simulink model "cascadecontrol"  (Simulink 6.0)
settings: Solver=ode45  StartTime=0.0  StopTime=1000  RelTol=1e-3
libraries: simulink_extras x3, simulink x1
settings Model: LastModifiedBy=lenovo

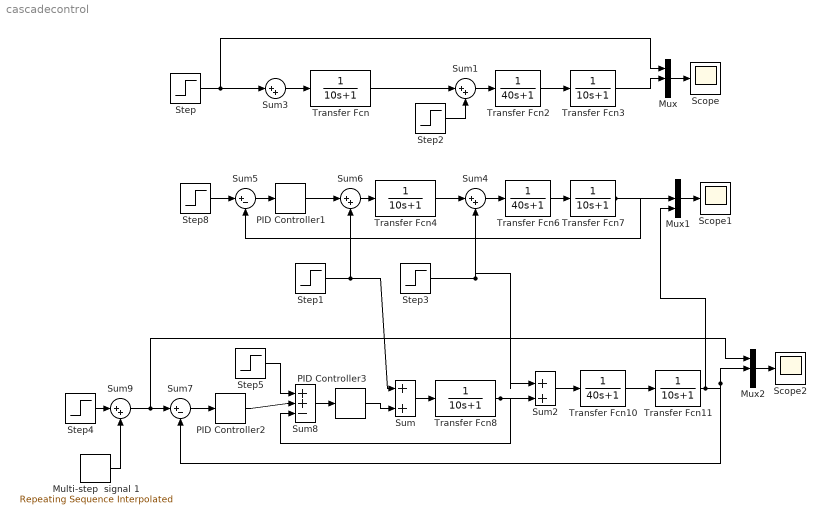
== system cascadecontrol ==
  Multi-step  signal 1 : simulink/Sources/Repeating Sequence Interpolated  OutValues=[1 2 1.5 1 1.5].'  TimeValues=[0 28 55 80 100]*10.'  LookUpMeth=Use Input Below  tsamp=1  OutputDataTypeScalingMode=Specify via dialog  OutDataType=float('double')  OutScaling=2^-10
  Mux : Mux  Inputs=3
  Mux1 : Mux  Inputs=3
  Mux2 : Mux  Inputs=3
  PID Controller1 : simulink_extras/Additional Linear/PID Controller  P=4  I=0.05  D=20
  PID Controller2 : simulink_extras/Additional Linear/PID Controller  P=10  I=0.15  D=45
  PID Controller3 : simulink_extras/Additional Linear/PID Controller  P=1.5  I=0  D=0
  Scope : Scope
  Scope1 : Scope
  Scope2 : Scope
      settings: SaveName=ScopeData2
  Step : Step  Time=0  SampleTime=0
  Step{1..5,8} (6 alike) : Step  Time=0  After=0  SampleTime=0
  Sum{,1..4,6,9} (7 alike) : Sum  Inputs=|++
  Sum5 : Sum  Inputs=|+-
  Sum7 : Sum  Inputs=|+-
  Sum8 : Sum  Inputs=|++-
  Transfer Fcn{,3..4,7..8,11} (6 alike) : TransferFcn  Denominator=[10 1]
  Transfer Fcn10 : TransferFcn  Denominator=[40 1]
  Transfer Fcn2 : TransferFcn  Denominator=[40 1]
  Transfer Fcn6 : TransferFcn  Denominator=[40 1]
  wires:
  Step/1 -> Mux/1, Sum3/1
  Transfer Fcn/1 -> Sum1/1
  Sum1/1 -> Transfer Fcn2/1
  Transfer Fcn3/1 -> Mux/2
  Mux/1 -> Scope/1
  Transfer Fcn2/1 -> Transfer Fcn3/1
  Sum5/1 -> PID Controller1/1
  PID Controller1/1 -> Sum6/1
  Sum4/1 -> Transfer Fcn6/1
  Transfer Fcn7/1 -> Sum5/2, Mux1/2
  Mux1/1 -> Scope1/1
  Sum6/1 -> Transfer Fcn4/1
  Transfer Fcn6/1 -> Transfer Fcn7/1
  Step2/1 -> Sum1/2
  Sum3/1 -> Transfer Fcn/1
  Step3/1 -> Sum4/2, Sum2/1
  Sum7/1 -> PID Controller2/1
  PID Controller2/1 -> Sum8/2
  Transfer Fcn11/1 -> Mux2/2, Sum7/2, Mux1/3
  Mux2/1 -> Scope2/1
  Sum8/1 -> PID Controller3/1
  Transfer Fcn10/1 -> Transfer Fcn11/1
  Step5/1 -> Sum8/1
  Step4/1 -> Sum9/1
  Sum9/1 -> Sum7/1, Mux2/1
  Transfer Fcn4/1 -> Sum4/1
  ? -> Sum3/2
  Sum/1 -> Transfer Fcn8/1
  PID Controller3/1 -> Sum/2
  Transfer Fcn8/1 -> Sum8/3, Sum2/2
  Sum2/1 -> Transfer Fcn10/1
  Multi-step  signal 1/1 -> Sum9/2
  Step8/1 -> Sum5/1
  Step1/1 -> Sum6/2, Sum/1
